simulink subsystem "PlannerMinJerk"  (R2025a)
settings: Solver=VariableStepAuto  StartTime=0.0  StopTime=10.0  RelTol=1e-3
undefined symbols (not defined in the file): Param_Planner_MinJerk_ReactionTime
libraries: arsenal x3
settings Model: DataDictionary=neck_mk3.sldd  EnableAccessToBaseWorkspace=off  Creator=upattacini  LastModifiedBy=upattacini
settings RTWCC: GPUComputeCapability=3.5

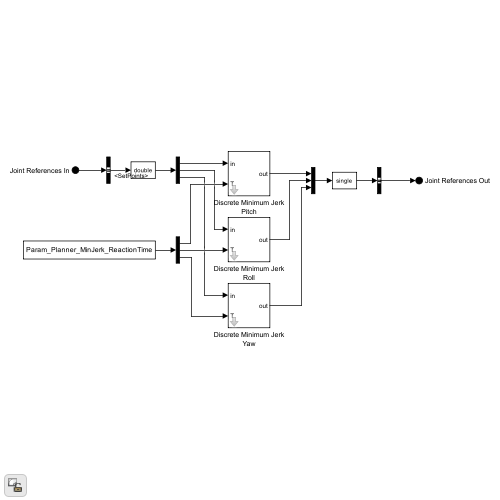
[thumbnail: Simulink's stored preview of the top-level diagram]
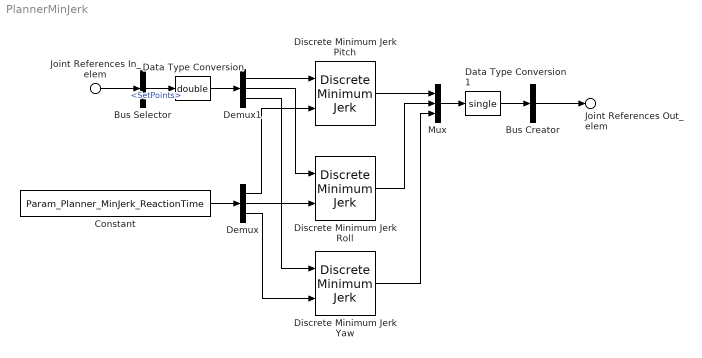
== system PlannerMinJerk ==
  Joint References In_elem : Inport  PortName=Joint References In
  Bus Creator : BusCreator  Inputs=1  OutDataTypeStr=Bus: Data_JointReferences  NonVirtualBus=on
      settings: InheritFromInputs=off
  Bus Selector : BusSelector  OutputSignals=SetPoints
  Constant : Constant  Value=Param_Planner_MinJerk_ReactionTime
  Data Type Conversion : DataTypeConversion  OutDataTypeStr=double  SaturateOnIntegerOverflow=off  RndMeth=Floor
  Data Type Conversion1 : DataTypeConversion  OutDataTypeStr=single  SaturateOnIntegerOverflow=off  RndMeth=Floor
  Demux : Demux  Outputs=3
  Demux1 : Demux  Outputs=3
  Discrete Minimum Jerk Pitch : arsenal/Filters/Discrete Minimum Jerk  Ts=0.001
      settings: SourceProductName=iCub Tech Arsenal
  Discrete Minimum Jerk Roll : arsenal/Filters/Discrete Minimum Jerk  Ts=0.001
      settings: SourceProductName=iCub Tech Arsenal
  Discrete Minimum Jerk Yaw : arsenal/Filters/Discrete Minimum Jerk  Ts=0.001
      settings: SourceProductName=iCub Tech Arsenal
  Mux : Mux  Inputs=3
  Joint References Out_elem : Outport  PortName=Joint References Out
  wires:
  Bus Creator/1 -> Joint References Out_elem/1
  Joint References In_elem/1 -> Bus Selector/1
  Bus Selector/1 -> Data Type Conversion/1  "<SetPoints>"
  Data Type Conversion1/1 -> Bus Creator/1
  Constant/1 -> Demux/1
  Data Type Conversion/1 -> Demux1/1
  Demux1/1 -> Discrete Minimum Jerk Pitch/1
  Discrete Minimum Jerk Pitch/1 -> Mux/1
  Mux/1 -> Data Type Conversion1/1
  Demux/2 -> Discrete Minimum Jerk Roll/2
  Demux/1 -> Discrete Minimum Jerk Pitch/2
  Demux1/2 -> Discrete Minimum Jerk Roll/1
  Demux/3 -> Discrete Minimum Jerk Yaw/2
  Demux1/3 -> Discrete Minimum Jerk Yaw/1
  Discrete Minimum Jerk Roll/1 -> Mux/2
  Discrete Minimum Jerk Yaw/1 -> Mux/3
